simulink model "hexa_tilted_ST"  (R2022b)
settings: Solver=ode1  StartTime=0.0  StopTime=tf  FixedStep=0.01  RelTol=1e-3
model workspace (MAT data in the model file):
  tf : Simulink.Parameter (value not decoded)
  tray0 = [0 0 0 0 0 0 0 0 5 0 0 0 ... (36 elements, 6x6)]
  tray1 = [0 0 0 0 0 0 0 0 5 0 0 0 ... (36 elements, 6x6)]
  tray2 = [0 0 0 0 0 0 2 0 5 0 0 0 ... (36 elements, 6x6)]
  tray3 = [0 0 0 0 0 0 2 0 5 0 0 0 ... (36 elements, 6x6)]
  tray4 = [0 0 0 0 0 0 2 0 5 0.15 0 0 ... (36 elements, 6x6)]
  tray5 = [0 0 0 0 0 0 0 0 5 0.15 0 0 ... (36 elements, 6x6)]
undefined symbols (not defined in the file or in its folder): smiData, X, Y, Z
libraries: sm_lib x50, robotcorelib x1, nesl_utility x1
(part 2 of 2)

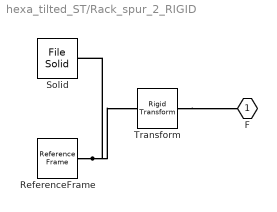
== system hexa_tilted_ST/Rack_spur_2_RIGID ==
  ReferenceFrame : sm_lib/Frames and Transforms/Reference Frame
  Solid : sm_lib/Body Elements/File Solid  ExtGeomFileName=Rack_spur_Metric - Rack-spur - rectangular 0.8M 14.5PA 3FW 10PH 75L---SAll_sldprt.STEP  UnitType=FromFile  ExtGeomFileUnits=m  StepReaderType=HEX  ExportConvexHullGeometry=off  InertiaType=Custom  Mass=smiData.Solid(3).mass  MassUnits=kg  CenterOfMass=smiData.Solid(3).CoM  CenterOfMassUnits=mm  MomentsOfInertia=smiData.Solid(3).MoI  MomentsOfInertiaUnits=kg*mm^2  ProductsOfInertia=smiData.Solid(3).PoI  ProductsOfInertiaUnits=kg*mm^2  BasedOnType=DensityFromFile  Density=1000  DensityUnits=kg/m^3  DoExposeReferenceFrame=on  SerializedFrames=<Frames/>  GraphicType=FromGeometry  MarkerShape=Sphere  MarkerSize=10  GraphicVisPropType=SimpleVisualProperties  GraphicDiffuseColor=smiData.Solid(3).color  GraphicSpecularColor=[0.5 0.5 0.5 1.0]  GraphicAmbientColor=[0.15 0.15 0.15 1.0]  GraphicEmissiveColor=[0.0 0.0 0.0 1.0]  GraphicShininess=75  GraphicOpacity=smiData.Solid(3).opacity
  Transform : sm_lib/Frames and Transforms/Rigid Transform  TranslationMethod=Cartesian  TranslationStandardOffset=0  TranslationLengthUnit=mm  TranslationStandardAxis=+Z  TranslationCartesianOffset=smiData.RigidTransform(4).translation  TranslationROffset=0  TranslationROffsetUnits=m  TranslationZOffset=0  TranslationZOffsetUnits=m  TranslationThetaOffset=0  TranslationThetaOffsetUnits=deg  RotationMethod=ArbitraryAxis  RotationAngleUnits=rad  RotationStandardAxis=+Z  RotationAngle=smiData.RigidTransform(4).angle  RotationArbitraryAxis=smiData.RigidTransform(4).axis  FollAlignAxisA=+X  BaseAlignAxisA=+Y  FollAlignAxisB=+Y  BaseAlignAxisB=+Z  RotationSequenceAxes=FollowerAxes  RotationSequence=XYX  RotationSequenceAngles=[0 0 0]  RotationSequenceAnglesUnits=deg  RotationMatrix=[1 0 0; 0 1 0; 0 0 1]  Quaternion=[1 0 0 0]
  F : PMIOPort  Side=Left
  connections:
  Solid/RConn1 -- ReferenceFrame/RConn1 -- Transform/LConn1
  Transform/RConn1 -- F/RConn1

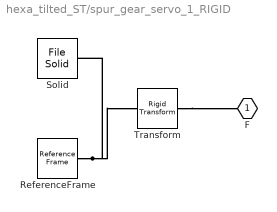
== system hexa_tilted_ST/spur_gear_servo_1_RIGID ==
  ReferenceFrame : sm_lib/Frames and Transforms/Reference Frame
  Solid : sm_lib/Body Elements/File Solid  ExtGeomFileName=spur_gear_servo_Metric - Spur gear 0.8M 36T 14.5PA 5FW ---S36N75H50L20N_sldprt.STEP  UnitType=FromFile  ExtGeomFileUnits=m  StepReaderType=HEX  ExportConvexHullGeometry=off  InertiaType=Custom  Mass=smiData.Solid(4).mass  MassUnits=kg  CenterOfMass=smiData.Solid(4).CoM  CenterOfMassUnits=mm  MomentsOfInertia=smiData.Solid(4).MoI  MomentsOfInertiaUnits=kg*mm^2  ProductsOfInertia=smiData.Solid(4).PoI  ProductsOfInertiaUnits=kg*mm^2  BasedOnType=DensityFromFile  Density=1000  DensityUnits=kg/m^3  DoExposeReferenceFrame=on  SerializedFrames=<Frames/>  GraphicType=FromGeometry  MarkerShape=Sphere  MarkerSize=10  GraphicVisPropType=SimpleVisualProperties  GraphicDiffuseColor=smiData.Solid(4).color  GraphicSpecularColor=[0.5 0.5 0.5 1.0]  GraphicAmbientColor=[0.15 0.15 0.15 1.0]  GraphicEmissiveColor=[0.0 0.0 0.0 1.0]  GraphicShininess=75  GraphicOpacity=smiData.Solid(4).opacity
  Transform : sm_lib/Frames and Transforms/Rigid Transform  TranslationMethod=Cartesian  TranslationStandardOffset=0  TranslationLengthUnit=mm  TranslationStandardAxis=+Z  TranslationCartesianOffset=smiData.RigidTransform(6).translation  TranslationROffset=0  TranslationROffsetUnits=m  TranslationZOffset=0  TranslationZOffsetUnits=m  TranslationThetaOffset=0  TranslationThetaOffsetUnits=deg  RotationMethod=ArbitraryAxis  RotationAngleUnits=rad  RotationStandardAxis=+Z  RotationAngle=smiData.RigidTransform(6).angle  RotationArbitraryAxis=smiData.RigidTransform(6).axis  FollAlignAxisA=+X  BaseAlignAxisA=+Y  FollAlignAxisB=+Y  BaseAlignAxisB=+Z  RotationSequenceAxes=FollowerAxes  RotationSequence=XYX  RotationSequenceAngles=[0 0 0]  RotationSequenceAnglesUnits=deg  RotationMatrix=[1 0 0; 0 1 0; 0 0 1]  Quaternion=[1 0 0 0]
  F : PMIOPort  Side=Left
  connections:
  Solid/RConn1 -- ReferenceFrame/RConn1 -- Transform/LConn1
  Transform/RConn1 -- F/RConn1

== matlab function hexa_tilted_ST/ST Constants ==
  data: unused input; lambda output; alpha output; c output; b output
function [lambda, alpha, c, b] = fcn(~)

% valores de lambda > 0
lambda = [25; 25; 25; 0.25; 0.25; 25];

% valores de K > 0
%K = [7.5; 7.5; 15; 5; 5; 5];

C_st = [25; 25; 25; 25; 25; 25];

c = 1.5 * sqrt(C_st);

b = 1.1 * C_st;

% valores de 0 < alpha < 1  
alpha = [0.5; 0.5; 0.5; 0.5; 0.5; 0.5];

== matlab function hexa_tilted_ST/Constants Functions ==
  data: Phi output; Rib output; Fg output; pose input; M output; M_inv output; allo output; v input
function [Phi, Rib, Fg, M, M_inv, allo] = fcn(pose, v)

%% system constants
pi = 3.141592;
m = 2.0; %5 mass 2.2 kg
l = 0.25; % length m
g = 9.81; % gravity m/s²
Jxx =  24778420.82/(1000*1000000); % kg m²
Jyy = 42217933.96/(1000*1000000); % kg m²
Jzz = 23948304.24/(1000*1000000); % kg m²
kT = 0.000006975938113;
kQ = 0.000118290418538;

%% Phi matrix calculation
uu = v(1);
vv = v(2);
ww = v(3);
pp = v(4);
qq = v(5);
rr = v(6);


Phi = [0, -rr, qq, 0, -ww, vv;
        rr, 0, -pp , ww, 0, -uu;
        -qq, pp, 0,  -vv, uu, 0;
        0, 0, 0, 0, -rr, qq; 
        0, 0, 0, rr, 0, -pp;
        0, 0, 0, -qq, pp, 0];

%% Rib matrix calculation

roll = pose(4);
pitch = pose(5);
yaw = pose(6);

Rib = [cos(yaw)*cos(pitch), -cos(roll)*sin(yaw) + cos(yaw)*sin(roll)*sin(pitch), sin(roll)*sin(yaw) + cos(roll)*cos(yaw)*sin(pitch), 0, 0, 0;
       cos(pitch)*sin(yaw), cos(roll)*cos(yaw) + sin(yaw)*sin(pitch)*sin(roll), -cos(yaw)*sin(roll) + sin(yaw)*sin(pitch)*cos(roll), 0, 0, 0;
       -sin(pitch), cos(pitch)*sin(roll), cos(pitch)*cos(roll), 0, 0, 0;
       0, 0, 0, 1, sin(roll)*tan(pitch), cos(roll)*tan(pitch);
       0, 0, 0, 0, cos(roll), -sin(roll);
       0, 0, 0, 0, sin(roll)/cos(pitch), cos(roll)/cos(pitch)];

%% Fg matrix calculation

Fg = [m*g*sin(pitch);
      -m*g*cos(pitch)*sin(roll);
      -m*g*cos(pitch)*cos(roll);
      0;
      0;
      0];

M = [m, 0, 0, 0, 0, 0;
    0, m, 0, 0, 0, 0;
    0, 0, m, 0, 0, 0;
    0, 0, 0, Jxx, 0, 0;
    0, 0, 0, 0, Jyy, 0;
    0, 0, 0, 0, 0, Jzz];

M_inv = inv(M);

alpha = [pi/6; -pi/6; -pi/2; -5*pi/6; 5*pi/6; pi/2];

varphi = pi/9;

%% tilted rotors matrix allocation

m11 = -kT*cos(alpha(1))*sin(varphi);
m21 = kT*sin(alpha(1))*sin(varphi);
m31 = kT*cos(varphi);
m41 = cos(alpha(1))*(l*kT*cos(varphi) - kQ*sin(varphi));
m51 = sin(alpha(1))*(-l*kT*cos(varphi) + kQ*sin(varphi));
m61 = l*kT*sin(varphi) + kQ*cos(varphi);

m12 = kT*cos(alpha(2))*sin(varphi);
m22 = -kT*sin(alpha(2))*sin(varphi);
m32 = m31;
m42 = cos(alpha(2))*(l*kT*cos(varphi) - kQ*sin(varphi));
m52 = sin(alpha(2))*(-l*kT*cos(varphi) + kQ*sin(varphi));
m62 = -l*kT*sin(varphi) - kQ*cos(varphi);

m13 = kT*cos(alpha(3))*sin(varphi);
m23 = kT*sin(alpha(3))*sin(varphi);
m33 = m31;
m43 = cos(alpha(3))*(l*kT*cos(varphi) + kQ*sin(varphi));
m53 = sin(alpha(3))*(-l*kT*cos(varphi) + kQ*sin(varphi));
m63 = l*kT*sin(varphi) + kQ*cos(varphi);

m14 = kT*cos(alpha(4))*sin(varphi);
m24 = -kT*sin(alpha(4))*sin(varphi);
m34 = m31;
m44 = cos(alpha(4))*(l*kT*cos(varphi) - kQ*sin(varphi));
m54 = sin(alpha(4))*(-l*kT*cos(varphi) + kQ*sin(varphi));
m64 = -l*kT*sin(varphi) - kQ*cos(varphi);

m15 = -kT*cos(alpha(5))*sin(varphi);
m25 = kT*sin(alpha(5))*sin(varphi);
m35 = m31;
m45 = cos(alpha(5))*(l*kT*cos(varphi) - kQ*sin(varphi));
m55 = sin(alpha(5))*(-l*kT*cos(varphi) + kQ*sin(varphi));
m65 = l*kT*sin(varphi) + kQ*cos(varphi);

m16 = kT*cos(alpha(6))*sin(varphi);
m26 = -kT*sin(alpha(6))*sin(varphi);
m36 = m31;
m46 = cos(alpha(6))*(l*kT*cos(varphi) + kQ*sin(varphi));
m56 = sin(alpha(6))*(-l*kT*cos(varphi) + kQ*sin(varphi));
m66 = -l*kT*sin(varphi) - kQ*cos(varphi);

allo = [m11, m12, m13, m14, m15, m16;
        m21, m22, m23, m24, m25, m26;
        m31, m32, m33, m34, m35, m36;
        m41, m42, m43, m44, m45, m46;
        m51, m52, m53, m54, m55, m56;
        m61, m62, m63, m64, m65, m66];

allo = inv(allo);
